simulink model "Final_part"  (R2016a)
settings: Solver=VariableStepAuto  StartTime=0.0  StopTime=15  RelTol=1e-3
libraries: fl_lib x19, nesl_utility x9, elec_lib x3, simulink x1
settings Model: Creator=SD  LastModifiedBy=SD

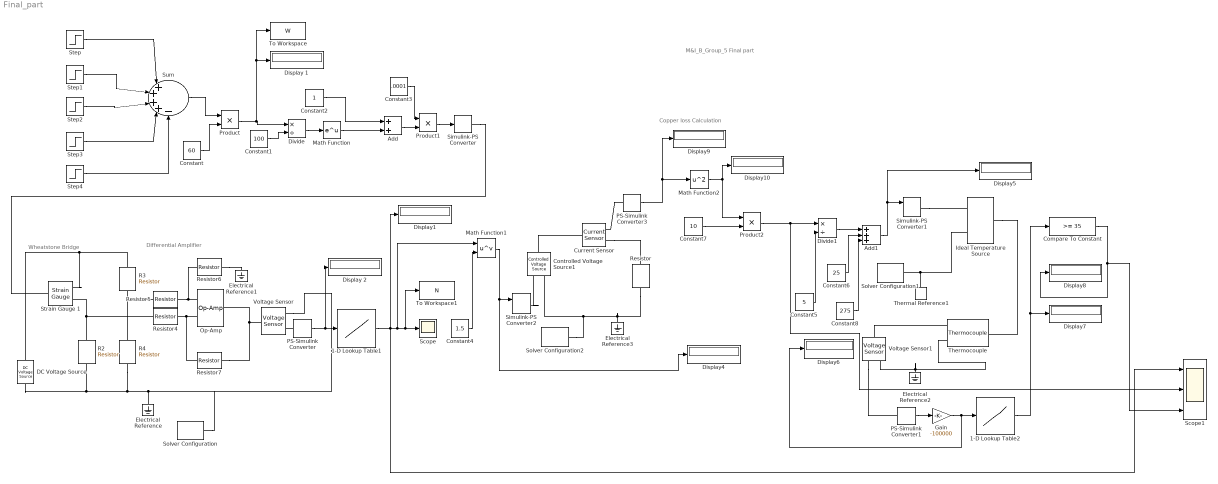
== system Final_part ==
  note: M&I_B_Group_5 Final part
  note: Copper loss Calculation
  note: Wheatstone Bridge
  note: Differential Amplifier
  1-D Lookup Table1 : Lookup_n-D  NumberOfTableDimensions=1  BreakpointsForDimension1=[.000403 .001006 .00174 .005334 .01712 ]  Table=[1 3 4 6 8 ]  InternalRulePriority=Speed  RndMeth=Simplest  InputSameDT=on
  1-D Lookup Table2 : Lookup_n-D  NumberOfTableDimensions=1  BreakpointsForDimension1=|  Table=|  InternalRulePriority=Speed  RndMeth=Simplest  InputSameDT=on
      BreakpointsForDimension1=|
      | [5.13
      | 5.43
      | 6.00
      | 6.95
      | 8.32
      | 10.20
      | 15.52
      | 22.76
      | 
      |  ]
      Table=|
      | [25.16
      | 25.54
      | 26.88
      | 27.50
      | 29.32
      | 31.86
      | 39.58
      | 51.62
      | ]
  Add : Sum
  Add1 : Sum  Inputs=+++
  Compare To Constant : simulink/Logic and Bit Operations/Compare To Constant  relop=>=  const=35  OutDataTypeStr=boolean
  Constant : Constant  Value=60
  Constant1 : Constant  Value=100
  Constant2 : Constant
  Constant3 : Constant  Value=.0001
  Constant4 : Constant  Value=1.5
  Constant5 : Constant  Value=5
  Constant6 : Constant  Value=25
  Constant7 : Constant  Value=10
  Constant8 : Constant  Value=275
  Controlled Voltage Source1 : fl_lib/Electrical/Electrical Sources/Controlled Voltage Source
  Current Sensor : fl_lib/Electrical/Electrical Sensors/Current Sensor
  DC Voltage Source : elec_lib/Additional Components/SPICE-Compatible Components/Sources/DC Voltage Source  DC=10 V
  Display 1 : Display
  Display 2 : Display
  Display{1,4..10} (8 alike) : Display
  Divide : Product  Inputs=*/
  Divide1 : Product  Inputs=*/  SaturateOnIntegerOverflow=on  RndMeth=Zero
  Electrical Reference{,1..3} (4 alike) : fl_lib/Electrical/Electrical Elements/Electrical Reference
  Gain : Gain  Gain=-100000
  Ideal Temperature Source : fl_lib/Thermal/Thermal Sources/Ideal Temperature Source
  Math Function : Math  SaturateOnIntegerOverflow=on
  Math Function1 : Math  Operator=pow  SaturateOnIntegerOverflow=on
      settings: LockScale=on
  Math Function2 : Math  Operator=square  SaturateOnIntegerOverflow=on
  Op-Amp : fl_lib/Electrical/Electrical Elements/Op-Amp  outI_specify=off  outI_priority=High  outI=0 A
  PS-Simulink Converter : nesl_utility/PS-Simulink Converter  PhysicalDomain=network_engine_domain  SubClassName=ps_output  LeftPortType=input  RightPortType=output  PseudoPeriodic=off  Frequencies=[]  Unit=1  AffineConversion=off
  PS-Simulink Converter1 : nesl_utility/PS-Simulink Converter  PhysicalDomain=network_engine_domain  SubClassName=ps_output  LeftPortType=input  RightPortType=output  PseudoPeriodic=off  Frequencies=[]  Unit=1  AffineConversion=off
  PS-Simulink Converter3 : nesl_utility/PS-Simulink Converter  PhysicalDomain=network_engine_domain  SubClassName=ps_output  LeftPortType=input  RightPortType=output  PseudoPeriodic=off  Frequencies=[]  Unit=1  AffineConversion=off
  Product : Product
  Product1 : Product
  Product2 : Product
  "R2 " : fl_lib/Electrical/Electrical Elements/Resistor  R=100 Ohm  i_specify=off  i_priority=High  i=0 A  v_specify=off  v_priority=High  v=0 V
  R3 : fl_lib/Electrical/Electrical Elements/Resistor  R=100 Ohm  i_specify=off  i_priority=High  i=0 A  v_specify=off  v_priority=High  v=0 V
  "R4 " : fl_lib/Electrical/Electrical Elements/Resistor  R=100 Ohm  i_specify=off  i_priority=High  i=0 A  v_specify=off  v_priority=High  v=0 V
  Resistor : fl_lib/Electrical/Electrical Elements/Resistor  R=10 Ohm  i_specify=off  i_priority=None  i=0 A  v_specify=off  v_priority=None  v=0 V
  Resistor{4..7} (4 alike) : fl_lib/Electrical/Electrical Elements/Resistor  R=10 Ohm  i_specify=off  i_priority=High  i=0 A  v_specify=off  v_priority=High  v=0 V
  Scope : Scope
  Scope1 : Scope  NumInputPorts=3
  Simulink-PS Converter : nesl_utility/Simulink-PS Converter  PhysicalDomain=network_engine_domain  SubClassName=ps_input  LeftPortType=input  RightPortType=output  PseudoPeriodic=off  Frequencies=[]  NoiseDistribution=none  NoiseParameters=[]  Unit=1  AffineConversion=off  InputFiltering=off  SimscapeFilterOrder=1  InputFilterTimeConstant=0.001  UdotUserProvided=1
  Simulink-PS Converter1 : nesl_utility/Simulink-PS Converter  PhysicalDomain=network_engine_domain  SubClassName=ps_input  LeftPortType=input  RightPortType=output  PseudoPeriodic=off  Frequencies=[]  NoiseDistribution=none  NoiseParameters=[]  Unit=1  AffineConversion=off  InputFiltering=derivs  SimscapeFilterOrder=1  InputFilterTimeConstant=0.001  UdotUserProvided=1
  Simulink-PS Converter2 : nesl_utility/Simulink-PS Converter  PhysicalDomain=network_engine_domain  SubClassName=ps_input  LeftPortType=input  RightPortType=output  PseudoPeriodic=off  Frequencies=[]  NoiseDistribution=none  NoiseParameters=[]  Unit=1  AffineConversion=off  InputFiltering=derivs  SimscapeFilterOrder=1  InputFilterTimeConstant=0.001  UdotUserProvided=1
  Solver Configuration : nesl_utility/Solver Configuration  PhysicalDomain=network_engine_domain  SubClassName=solver  LeftPortType=input  RightPortType=generic  Accelerate=off  Tones=[]  Harmonics=[]  SimulateNoise=off  Profile=off  UseLocalSampling=off  EnableSwitchedLinearOptims=on  FrequencyDomain=off  UseCCode=off  RelTol=0.001  AbsTol=1e-06  MinStep=1e-09  ToWorkspace=off  RevertToSquareIcSolve=off  NumHomotopyIterations=100  PhasorMode=off  PhasorModeNumHarmonics=1  OverrideAbsTol=off  DoDC=off  ResidualTolerance=1e-09  UseLocalSolver=off  LocalSolverChoice=NE_BACKWARD_EULER_ADVANCER  LocalSolverSampleTime=0.001  DoFixedCost=off  MaxNonlinIter=3  MaxModeIter=2  LinearAlgebra=Sparse  DelaysMemoryBudget=1024  AutomaticFiltering=on  FilteringTimeConstant=0.001
  Solver Configuration1 : nesl_utility/Solver Configuration  PhysicalDomain=network_engine_domain  SubClassName=solver  LeftPortType=input  RightPortType=generic  Accelerate=off  Tones=[]  Harmonics=[]  SimulateNoise=off  Profile=off  UseLocalSampling=off  EnableSwitchedLinearOptims=on  FrequencyDomain=off  UseCCode=off  RelTol=0.001  AbsTol=1e-06  MinStep=1e-09  ToWorkspace=off  RevertToSquareIcSolve=off  NumHomotopyIterations=100  PhasorMode=off  PhasorModeNumHarmonics=1  OverrideAbsTol=off  DoDC=off  ResidualTolerance=1e-09  UseLocalSolver=off  LocalSolverChoice=NE_BACKWARD_EULER_ADVANCER  LocalSolverSampleTime=0.001  DoFixedCost=off  MaxNonlinIter=3  MaxModeIter=2  LinearAlgebra=Sparse  DelaysMemoryBudget=1024  AutomaticFiltering=on  FilteringTimeConstant=0.001
  Solver Configuration2 : nesl_utility/Solver Configuration  PhysicalDomain=network_engine_domain  SubClassName=solver  LeftPortType=input  RightPortType=generic  Accelerate=off  Tones=[]  Harmonics=[]  SimulateNoise=off  Profile=off  UseLocalSampling=off  EnableSwitchedLinearOptims=on  FrequencyDomain=off  UseCCode=off  RelTol=0.001  AbsTol=1e-06  MinStep=1e-09  ToWorkspace=off  RevertToSquareIcSolve=off  NumHomotopyIterations=100  PhasorMode=off  PhasorModeNumHarmonics=1  OverrideAbsTol=off  DoDC=off  ResidualTolerance=1e-09  UseLocalSolver=off  LocalSolverChoice=NE_BACKWARD_EULER_ADVANCER  LocalSolverSampleTime=0.001  DoFixedCost=off  MaxNonlinIter=3  MaxModeIter=2  LinearAlgebra=Sparse  DelaysMemoryBudget=1024  AutomaticFiltering=on  FilteringTimeConstant=0.001
  Step : Step  Time=2  SampleTime=0
  Step1 : Step  Time=4  After=2  SampleTime=0
  Step2 : Step  Time=6  After=3  SampleTime=0
  Step3 : Step  Time=8  After=2  SampleTime=0
  Step4 : Step  Time=10  After=4  SampleTime=0
  Strain Gauge 1 : elec_lib/Sensors/Strain Gauge  R=100 Ohm  K=2
  Sum : Sum  Inputs=|++++-
  Thermal Reference1 : fl_lib/Thermal/Thermal Elements/Thermal Reference
  Thermocouple : elec_lib/Sensors/Thermocouple  Cvec=[ 0 0.0054031 1.2593e-5 -2.3248e-8 3.2203e-11 -3.3147e-14 2.5574e-17 -1.2507e-20 2.7144e-24 ]  T0=0 degC  tc=1 s  K_d=0.001 W/K  init_temp=25 degC
  To Workspace : ToWorkspace  VariableName=W  SampleTime=-1
  To Workspace1 : ToWorkspace  VariableName=N  SampleTime=-1
  Voltage Sensor : fl_lib/Electrical/Electrical Sensors/Voltage Sensor
  Voltage Sensor1 : fl_lib/Electrical/Electrical Sensors/Voltage Sensor
  wires:
  Step/1 -> Sum/1
  Sum/1 -> Product/1
  Constant/1 -> Product/2
  Product1/1 -> Simulink-PS Converter/1
  Constant3/1 -> Product1/1
  Add/1 -> Product1/2
  Math Function/1 -> Add/2
  Constant2/1 -> Add/1
  Divide/1 -> Math Function/1
  Product/1 -> Display 1/1, To Workspace/1, Divide/1
  PS-Simulink Converter/1 -> Display 2/1, 1-D Lookup Table1/1
  Constant1/1 -> Divide/2
  Step1/1 -> Sum/2
  Step2/1 -> Sum/3
  Step3/1 -> Sum/4
  1-D Lookup Table1/1 -> Scope1/1, To Workspace1/1, Scope/1, Math Function1/1, Display1/1
  Step4/1 -> Sum/5
  Gain/1 -> 1-D Lookup Table2/1, Display6/1
  PS-Simulink Converter3/1 -> Math Function2/1, Display9/1
  Math Function1/1 -> Display4/1, Simulink-PS Converter2/1
  Product2/1 -> Scope1/2, Divide1/1
  Constant5/1 -> Divide1/2
  Divide1/1 -> Add1/1
  Constant6/1 -> Add1/2
  Add1/1 -> Simulink-PS Converter1/1, Display5/1
  PS-Simulink Converter1/1 -> Gain/1
  1-D Lookup Table2/1 -> Display7/1, Compare To Constant/1
  Compare To Constant/1 -> Display8/1, Scope1/3
  Constant4/1 -> Math Function1/2
  Constant7/1 -> Product2/2
  Math Function2/1 -> Product2/1, Display10/1
  Constant8/1 -> Add1/3
  connections:
  "R4 "/LConn1 -- R3/RConn1 -- Resistor5/LConn1
  "R2 "/LConn1 -- Resistor4/LConn1 -- Strain Gauge 1/RConn2
  "R2 "/RConn1 -- DC Voltage Source/RConn1 -- "R4 "/RConn1 -- Electrical Reference/LConn1 -- Voltage Sensor/RConn2 -- Solver Configuration/RConn1
  Resistor4/RConn1 -- Resistor7/LConn1 -- Op-Amp/LConn2
  Resistor6/LConn1 -- Resistor5/RConn1 -- Op-Amp/LConn1
  Resistor7/RConn1 -- Op-Amp/RConn1 -- Voltage Sensor/LConn1
  R3/LConn1 -- Strain Gauge 1/RConn1 -- DC Voltage Source/LConn1
  Simulink-PS Converter/RConn1 -- Strain Gauge 1/LConn1
  PS-Simulink Converter/LConn1 -- Voltage Sensor/RConn1
  Resistor6/RConn1 -- Electrical Reference1/LConn1
  Thermal Reference1/LConn1 -- Ideal Temperature Source/RConn2 -- Solver Configuration1/RConn1
  Voltage Sensor1/RConn2 -- Thermocouple/LConn2 -- Electrical Reference2/LConn1
  Controlled Voltage Source1/LConn1 -- Current Sensor/LConn1
  Electrical Reference3/LConn1 -- Resistor/RConn1 -- Solver Configuration2/RConn1 -- Controlled Voltage Source1/RConn2
  Simulink-PS Converter1/RConn1 -- Ideal Temperature Source/RConn1
  Simulink-PS Converter2/RConn1 -- Controlled Voltage Source1/RConn1
  Thermocouple/LConn1 -- Voltage Sensor1/LConn1
  Ideal Temperature Source/LConn1 -- Thermocouple/RConn1
  Voltage Sensor1/RConn1 -- PS-Simulink Converter1/LConn1
  Current Sensor/RConn2 -- Resistor/LConn1
  PS-Simulink Converter3/LConn1 -- Current Sensor/RConn1
